simulink model "gyroscope_2021"  (R2021a)
settings: Solver=VariableStepAuto  StartTime=0.0  StopTime=100  RelTol=1e-3
libraries: simulink x1
settings Model: Creator=juliaye  LastModifiedBy=yeyifan
settings DebuggingCC: UnconnectedInputMsg=none  UnconnectedOutputMsg=none  UnconnectedLineMsg=none
settings RTWCC: DLArmComputeVersion=20.02.1

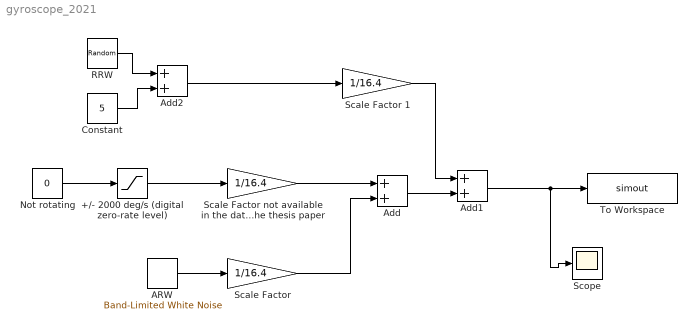
== system gyroscope_2021 ==
  +/- 2000 deg/s (digital zero-rate level) : Saturate  UpperLimit=2000  LowerLimit=-2000  LinearizeAsGain=off
  ARW : simulink/Sources/Band-Limited White Noise  Cov=[0.01^2]  Ts=1/100  seed=[23341]
  Add : Sum
  Add1 : Sum
  Add2 : Sum
  Constant : Constant  Value=5
  Not rotating : Constant  Value=0
  RRW : RandomNumber  Mean=0.01  Variance=0.001  SampleTime=0.1
  "Scale Factor " : Gain  Gain=1/16.4
  Scale Factor 1 : Gain  Gain=1/16.4
  Scale Factor not available in the datasheet taken from the thesis paper : Gain  Gain=1/16.4
  Scope : Scope
  To Workspace : ToWorkspace  VariableName=simout  SaveFormat=Timeseries  SampleTime=-1
  wires:
  Not rotating/1 -> +/- 2000 deg/s (digital zero-rate level)/1
  +/- 2000 deg/s (digital zero-rate level)/1 -> Scale Factor not available in the datasheet taken from the thesis paper/1
  Scale Factor not available in the datasheet taken from the thesis paper/1 -> Add/1
  ARW/1 -> "Scale Factor "/1
  "Scale Factor "/1 -> Add/2
  Add/1 -> Add1/2
  Scale Factor 1/1 -> Add1/1
  Add1/1 -> Scope/1, To Workspace/1
  RRW/1 -> Add2/1
  Constant/1 -> Add2/2
  Add2/1 -> Scale Factor 1/1
